simulink model "bldc_motor"  (R2019b)
settings: Solver=VariableStepAuto  StartTime=0.0  StopTime=4  RelTol=1e-8
InitFcn:
  | p = 46;
  | R = 0.15;
  | L= 0.0056;
  | Kf =0.001;
  | J = 0.01;
  | Ke = 1.3;
  | Kt = 0.972;
model workspace (MAT data in the model file):
  J = 0.1
  Ke = 1.278
  Kf = 0.001
  Kt = 0.9852
  L = 0.0056
  R = 0.15
  p = 46
settings Model: Creator=srikesh  LastModifiedBy=srikesh

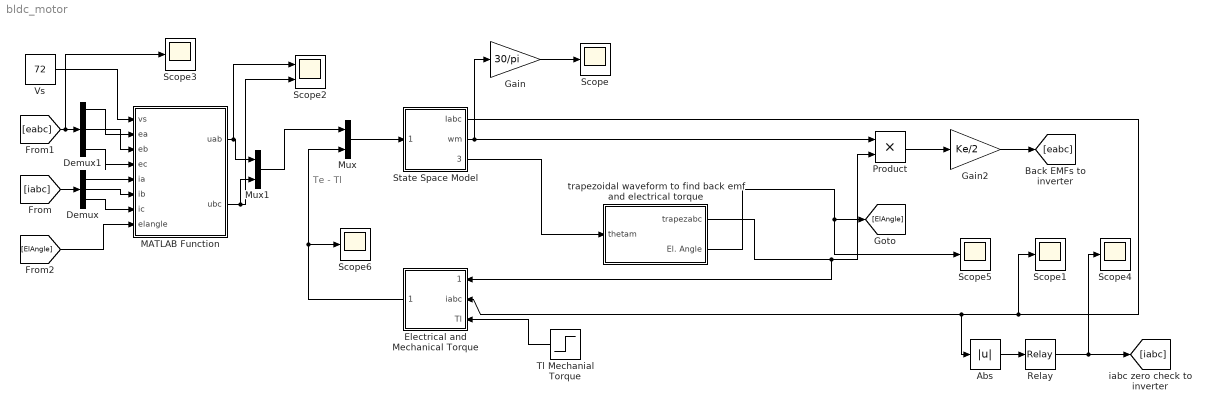
== system bldc_motor ==
  note: Te - Tl
  Abs : Abs
  Demux : Demux  Outputs=3
  Demux1 : Demux  Outputs=3
  Electrical and Mechanical Torque : Subsystem
  Gain : Gain  Gain=30/pi
  Gain2 : Gain  Gain=Ke/2
  MATLAB Function : MATLAB Function  TreatAsAtomicUnit=on
  Mux : Mux  Inputs=2
  Mux1 : Mux  Inputs=2
  "Product " : Product
  Relay : Relay
  Scope{,1,3..6} (6 alike) : Scope
  Scope2 : Scope  NumInputPorts=2
  "State Space Model " : Subsystem
  Tl Mechanial Torque : Step  Time=0  After=5  SampleTime=0
  "Vs " : Constant  Value=72
  "trapezoidal waveform to find back emf and electrical torque " : Subsystem
  wires:
  Mux/1 -> "State Space Model "/1("Input (u) ")
  "State Space Model "/1("Iabc ") -> Abs/1, Electrical and Mechanical Torque/2(iabc), Scope1/1
  "State Space Model "/2(wm) -> "Product "/1, Gain/1
  "Product "/1 -> Gain2/1
  Gain2/1 -> [eabc]
  "trapezoidal waveform to find back emf and electrical torque "/1(trapezabc) -> Electrical and Mechanical Torque/1("trapezabc "), "Product "/2
  "State Space Model "/3(thetam) -> "trapezoidal waveform to find back emf and electrical torque "/1("thetam ")
  Electrical and Mechanical Torque/1("Te - Tl ") -> Scope6/1, Mux/2
  [iabc] -> Demux/1
  [eabc] -> Scope3/1, Demux1/1
  Demux1/1 -> MATLAB Function/2(ea)
  Demux1/2 -> MATLAB Function/3(eb)
  Demux1/3 -> MATLAB Function/4(ec)
  Demux/1 -> MATLAB Function/5(ia)
  Demux/2 -> MATLAB Function/6(ib)
  Demux/3 -> MATLAB Function/7(ic)
  [ElAngle] -> MATLAB Function/8(elangle)
  MATLAB Function/1(uab) -> Scope2/1, Mux1/1
  MATLAB Function/2(ubc) -> Scope2/2, Mux1/2
  "Vs "/1 -> MATLAB Function/1(vs)
  Tl Mechanial Torque/1 -> Electrical and Mechanical Torque/3(Tl)
  Gain/1 -> Scope/1
  "trapezoidal waveform to find back emf and electrical torque "/2(El. Angle) -> Scope5/1, [ElAngle]
  Abs/1 -> Relay/1
  Relay/1 -> Scope4/1, [iabc]
  Mux1/1 -> Mux/1

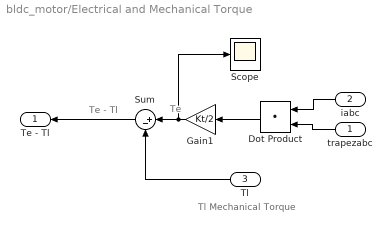
== system bldc_motor/Electrical and Mechanical Torque ==
  note: Te - Tl
  note: Te
  note: Tl Mechanical Torque
  "trapezabc " : Inport
  iabc : Inport  Port=2
  Tl : Inport  Port=3
  "Dot Product " : DotProduct  InputSameDT=on  OutDataTypeStr=Inherit: Inherit via internal rule
  Gain1 : Gain  Gain=Kt/2
  Scope : Scope
  Sum : Sum  Inputs=|+-
  "Te - Tl " : Outport
  wires:
  "Dot Product "/1 -> Gain1/1
  iabc/1 -> "Dot Product "/1
  Tl/1 -> Sum/2
  Sum/1 -> "Te - Tl "/1
  Gain1/1 -> Scope/1, Sum/1
  "trapezabc "/1 -> "Dot Product "/2

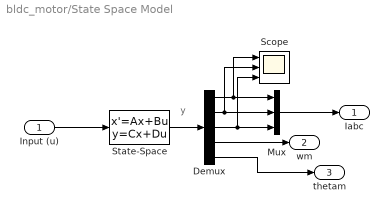
== system bldc_motor/State Space Model  ==
  note: y
  "Input (u) " : Inport
  Demux : Demux  Outputs=5
  Mux : Mux  Inputs=3
  Scope : Scope  NumInputPorts=3
  State-Space : StateSpace  A=[-R/L 0 0 0; 0 -R/L 0 0; 0 0 -Kf/J 0; 0 0 1 0]  B=[((2/3)*L) ((1/3)*L) 0; -((1/3)*L) ((1/3)*L) 0; 0 0 1/J; 0 0 0]  C=[1 0 0 0; 0 1 0 0; -1 -1 0 0; 0 0 1 0; 0 0 0 1]  D=[0 0 0; 0 0 0; 0 0 0; 0 0 0; 0 0 0]  InitialCondition=0
  "Iabc " : Outport
  wm : Outport  Port=2
  thetam : Outport  Port=3
  wires:
  State-Space/1 -> Demux/1
  "Input (u) "/1 -> State-Space/1
  Demux/2 -> Mux/2, Scope/2
  Mux/1 -> "Iabc "/1
  Demux/4 -> wm/1
  Demux/5 -> thetam/1
  Demux/1 -> Scope/1, Mux/1
  Demux/3 -> Scope/3, Mux/3

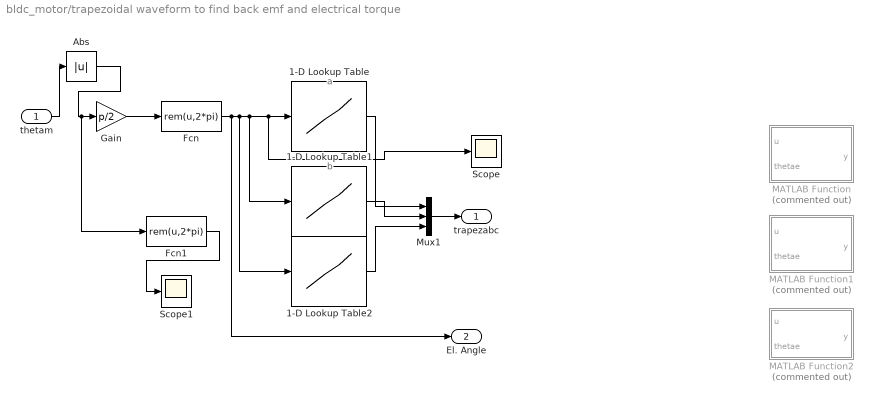
== system bldc_motor/trapezoidal waveform to find back emf and electrical torque  ==
  note: b
  note: a
  "thetam " : Inport
  1-D Lookup Table : Lookup_n-D  NumberOfTableDimensions=1  BreakpointsForDimension1=[0 2*pi/3 pi 5*pi/3 2*pi]  Table=[1 1 -1 -1 1]  InternalRulePriority=Speed  RndMeth=Simplest  InputSameDT=on
  1-D Lookup Table1 : Lookup_n-D  NumberOfTableDimensions=1  BreakpointsForDimension1=[0 pi/3 2*pi/3 4*pi/3 5*pi/3 2*pi]  Table=[-1 -1 1 1 -1 -1]  InternalRulePriority=Speed  RndMeth=Simplest  InputSameDT=on
  1-D Lookup Table2 : Lookup_n-D  NumberOfTableDimensions=1  BreakpointsForDimension1=[0 pi/3 pi 4*pi/3 2*pi]  Table=[1 -1 -1 1 1]  InternalRulePriority=Speed  RndMeth=Simplest  InputSameDT=on
  Abs : Abs
  Fcn : Fcn  Expr=rem(u,2*pi)
  Fcn1 : Fcn  Expr=rem(u,2*pi)
  Gain : Gain  Gain=p/2
  MATLAB Function : MATLAB Function  Commented=on  TreatAsAtomicUnit=on
  MATLAB Function1 : MATLAB Function  Commented=on  TreatAsAtomicUnit=on
  MATLAB Function2 : MATLAB Function  Commented=on  TreatAsAtomicUnit=on
  Mux1 : Mux  Inputs=3
  Scope : Scope
  Scope1 : Scope
  trapezabc : Outport
  El. Angle : Outport  Port=2
  wires:
  Gain/1 -> Fcn/1
  1-D Lookup Table1/1 -> Mux1/2
  Fcn/1 -> El. Angle/1, 1-D Lookup Table2/1, 1-D Lookup Table1/1, Scope/1, 1-D Lookup Table/1
  Mux1/1 -> trapezabc/1
  1-D Lookup Table/1 -> Mux1/1
  1-D Lookup Table2/1 -> Mux1/3
  Fcn1/1 -> Scope1/1
  "thetam "/1 -> Abs/1
  Abs/1 -> Fcn1/1, Gain/1

== matlab function bldc_motor/trapezoidal waveform to find back emf and electrical torque /MATLAB Function1 ==
  data: u input; y output; thetae input
function y = bfcn(u,thetae)
if((2*pi/3)<=u<(4*pi/3))
    y=1;
elseif((4*pi/3)<=u<(5*pi/3))
    y = 1-(6/pi)*(u-(2*pi/3));
elseif(((5*pi/3)<=u<(2*pi))||(0<=u<(pi/3)))
    y = -1;
elseif((pi/3)<=u<(2*pi/3))
    y = -1+(6/pi)*(u-(5*pi/3));
else 
    y = 1;
end
end

== matlab function bldc_motor/trapezoidal waveform to find back emf and electrical torque /MATLAB Function ==
  data: u input; y output; thetae input
function y = afcn(u,thetae)
if(0<=u<2*pi/3)
    y=1;
elseif((2*pi/3)<=u<pi)
    y = 1-(6/pi)*(u-(2*pi/3));
elseif(pi<=u<(5*pi/3))
    y = -1;
elseif((5*pi/3)<=u<(2*pi))
    y = -1+(6/pi)*(u-(5*pi/3));
else 
    y = 1;
end
end

== matlab function bldc_motor/trapezoidal waveform to find back emf and electrical torque /MATLAB Function2 ==
  data: u input; y output; thetae input
function y = cfcn(u,thetae)
if((4*pi/3)<=u<(2*pi))
    y=1;
elseif((0)<=u<(pi/3))
    y = 1-(6/pi)*(u-(2*pi/3));
elseif(((pi/3)<=u<(pi)))
    y = -1;
elseif(pi<=u<(4*pi/3))
    y = -1+(6/pi)*(u-(5*pi/3));
else
    y = 1;
end
end

== matlab function bldc_motor/MATLAB Function ==
  data: vs input; ea input; uab output; eb input; ec input; ia input; ib input; ic input; elangle input; ubc output
function [uab, ubc] = inver(vs, ea, eb, ec, ia, ib, ic, elangle)
    if(0<=elangle<(pi/3))
        if(ic~=0)
            uab = vs - ea + eb;
            ubc = -eb + ec;
        else
            uab = vs - ea + eb;
            ubc = 0.5*(-vs + ea - eb);
%         else
%             uab = 0;
%             ubc = 0;
        end
    elseif((pi/3)<=elangle<(2*pi/3))
        if(ib~=0)
            uab = -ea + eb;
            ubc = vs -eb + ec;
        else
            uab = 0.5*(vs - ea + ec);
            ubc = 0.5*(vs - ea + ec);
%         else
%             uab = 0;
%             ubc = 0;
        end
    elseif((2*pi/3)<=elangle<pi)
        if(ia~=0)
            uab = -vs - ea + eb;
            ubc = vs - eb + ec; 
        else
            uab = 0.5*(-vs + eb - ec);
            ubc = vs - eb + ec;
%         else
%             uab = 0;
%             ubc = 0;
        end
    elseif(pi<=elangle<(4*pi/3))
        if(ic~=0)
            uab = -vs - ea + eb;
            ubc = -eb + ec;
        else
            uab = -vs - ea + eb;
            ubc = 0.5*(vs + ea - eb);
%         else
%             uab = 0;
%             ubc = 0;
        end
    elseif((4*pi/3)<=elangle<(5*pi/3))
        if(ib~=0)
            uab = -ea + eb;
            ubc = -vs -eb + ec;
        else
            uab = 0.5*(-vs - ea + ec);
            ubc = 0.5*(-vs - ea + ec);
%         else
%             uab = 0;
%             ubc = 0;
        end
    elseif((5*pi/3)<=elangle<=(2*pi))
        if(ia~=0)
            uab = vs - ea + eb;
            ubc = -vs - eb + ec;
        else
            uab = 0.5*(vs + eb - ec);
            ubc = -vs - eb + ec;
%         else
%             uab = 0;
%             ubc = 0;
        end
    else 
        uab = 0;
        ubc = 0;
    end
end
